simulink library "ctl"  (R2024a)
settings: Solver=VariableStepAuto  StartTime=0.0  StopTime=10.0  RelTol=1e-3
undefined symbols (not defined in the file): deepc_params
libraries: otter_controllers x1
settings Model: Creator=mandicluka  LastModifiedBy=luka
settings RTWCC: GPUComputeCapability=3.5

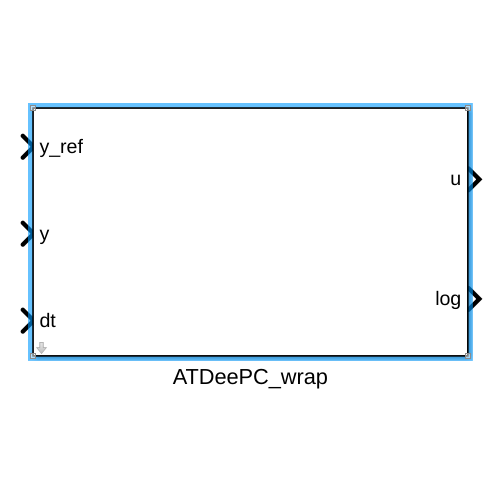
[thumbnail: Simulink's stored preview of the top-level diagram]
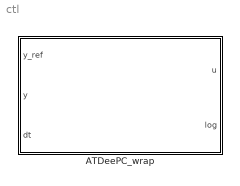
== system ctl ==
  ATDeePC_wrap : Subsystem  Tag=controller;  mask{params=deepc_params, trajectory_T=0, data=0, db_params=0, deepc_params=0}
      mask prompts: params "Parameter struct:"

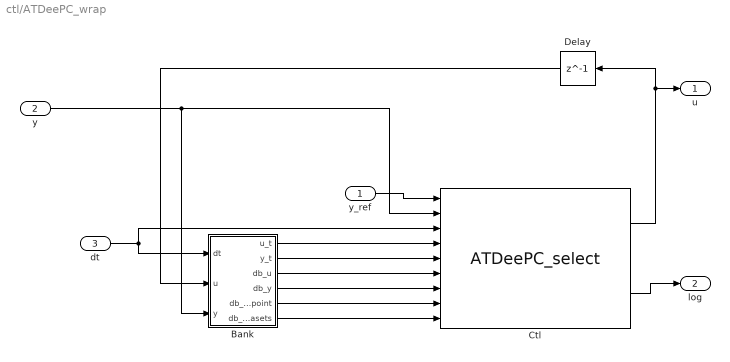
== system ctl/ATDeePC_wrap ==
  y_ref : Inport
  y : Inport  Port=2
  dt : Inport  Port=3
  Bank : MATLAB Function  TreatAsAtomicUnit=on
  Ctl : otter_controllers/ATDeePC_select  SystemSampleTime=-1  VariantActivationTime=update diagram  AllowFlexibleInterface=on  Latency=0  AutoFrameSizeCalculation=off
      link override ATDeePC1: params=params.deepc_params
  Delay : Delay  DelayLength=1
  u : Outport
  log : Outport  Port=2
  wires:
  Bank/6(db_num_datasets) -> Ctl/9
  Bank/5(db_endpoint) -> Ctl/8
  Bank/4(db_y) -> Ctl/7
  Bank/3(db_u) -> Ctl/6
  Bank/2(y_t) -> Ctl/5
  Bank/1(u_t) -> Ctl/4
  Delay/1 -> Bank/2(u)
  Ctl/2 -> log/1
  Ctl/1 -> u/1, Delay/1
  dt/1 -> Ctl/3, Bank/1(dt)
  y_ref/1 -> Ctl/1
  y/1 -> Ctl/2, Bank/3(y)

== matlab function ctl/ATDeePC_wrap/Bank ==
  settings: updateMethod=DISCRETE
  data: u_t output; y_t output; dt input; db_u output; u input; y input; db_params parameter; data parameter; db_y output; db_endpoint output; db_num_datasets output
function [u_t, y_t, db_u, db_y, db_endpoint, db_num_datasets] = fcn(dt, u, y, db_params, data)

    persistent t u_traj y_traj last_changed_t db_u_p db_y_p db_endpoint_p db_num_datasets_p    

    traj_len = data.T;
    if isempty(t)
        t = 0;
        last_changed_t = 0;
        db_num_datasets_p = db_params.num_datasets_in_bank;
        db_u_p = zeros(db_params.dataset_bank_size, data.T, data.m);
        db_y_p = zeros(db_params.dataset_bank_size, data.T, data.p);
        db_endpoint_p = zeros(db_params.dataset_bank_size, data.m);
        if db_num_datasets_p > 0
            db_u_p(end-db_num_datasets_p+1, :, :) = db_params.D_u;
            db_y_p(end-db_num_datasets_p+1, :, :) = db_params.D_y;
            db_endpoint_p(end-db_num_datasets_p+1, :, :) = db_params.end_point;
        end
        u_traj = zeros(traj_len, data.m);
        y_traj = zeros(traj_len, data.p);
    end

    t = t + dt;

    coder.extrinsic('trajectory_dataset'); % arx function not supported
    u_traj = circshift(u_traj, -1);
    y_traj = circshift(y_traj, -1);
    u_traj(end, :) = u(db_params.input_record_dims);
    y_traj(end, :) = y(db_params.output_record_dims);

    u_t = u_traj;
    y_t = y_traj;    
    
    
    [t, last_changed_t, db_u_p, db_y_p, db_endpoint_p, db_num_datasets_p, ...
       db_u, db_y, db_endpoint, db_num_datasets] = ...
          update_dataset_bank(t, last_changed_t, db_u_p, db_y_p, db_endpoint_p, db_num_datasets_p, dt, u_traj, y_traj, db_params, data);

end
